simulink model "elevation_techo_PLANT"  (R2022a)
settings: Solver=VariableStepAuto  StartTime=0.0  StopTime=100.0  RelTol=1e-4
undefined symbols (not defined in the file or in its folder): fix_conset, JLret, JMret, Kket, Kvet
libraries: slctrlblks x1
settings Model: Creator=ohadformanair  LastModifiedBy=ohadformanair
settings SolverCC: ZeroCrossAlgorithm=Adaptive
settings DebuggingCC: IgnoredZcDiagnostic=none

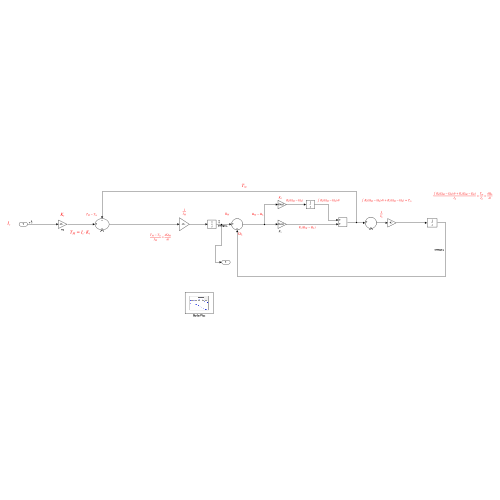
[thumbnail: Simulink's stored preview of the top-level diagram]
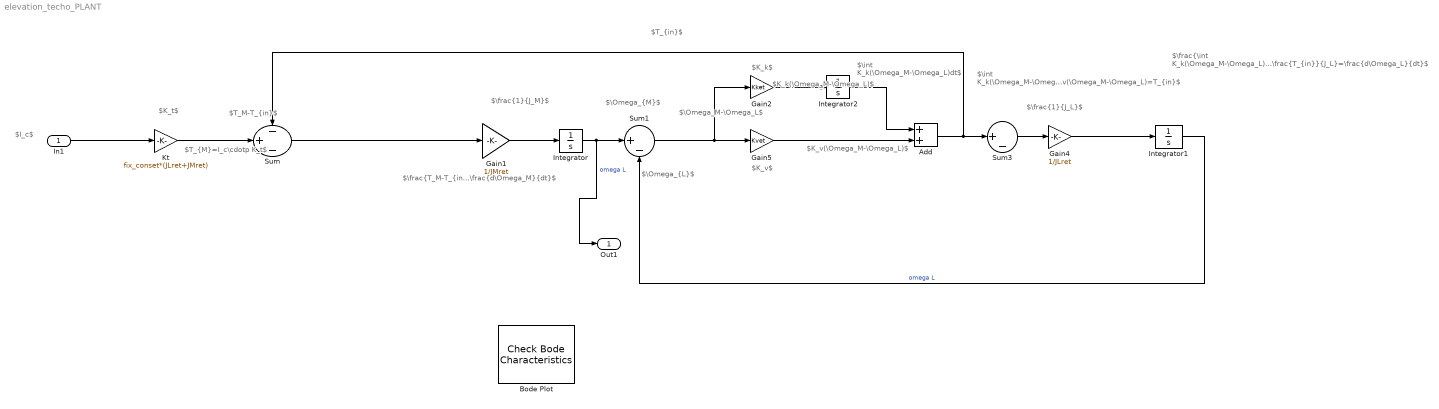
== system elevation_techo_PLANT ==
  note: $\Omega_{L}$
  note: $\frac{1}{J_L}$
  note: $K_v(\Omega_M-\Omega_L)$
  note: $T_{M}=I_c\cdotp K_t$
  note: $\frac{T_M-T_{in}}{J_M}=\frac{d\Omega_M}{dt}$
  note: $\int K_k(\Omega_M-\Omega_L)dt+K_v(\Omega_M-\Omega_L)=T_{in}$
  note: $I_c$
  note: $T_M-T_{in}$
  note: $K_k$
  note: $\Omega_M-\Omega_L$
  note: $\int K_k(\Omega_M-\Omega_L)dt$
  note: $K_k(\Omega_M-\Omega_L)$
  note: $\frac{1}{J_M}$
  note: $\frac{\int K_k(\Omega_M-\Omega_L)dt+K_v(\Omega_M-\Omega_L)}{J_L}=\frac{T_{in}}{J_L}=\frac{d\Omega_L}{dt}$
  note: $\Omega_{M}$
  note: $K_t$
  note: $K_v$
  note: $T_{in}$
  In1 : Inport
  Add : Sum
  Bode Plot : slctrlblks/Model Verification/Check Bode  Characteristics  InstantiateOnLoad=on  SaveOperatingPoints=off  LinearizationIOs={'/In1', 1, 'in', 'off', '';'/Integrator', 1, 'out', 'off', ''}  LinearizeAt=SnapshotTimes  SnapshotTimes=[0]  TriggerType=rising  SampleTime=auto  RateConversionMethod=zoh  PreWarpFreq=10  UseExactDelayModel=off  UseFullBlockNameLabels=off  UseBusSignalLabels=off  enabled=on  stopWhenAssertionFail=off  export=off  ViewDlgPos=[100 200 510 390]  OpenViewOnLoad=off  LaunchViewOnOpen=off  FrequencyUnits=Hz  MagnitudeUnits=dB  PhaseUnits=deg  TimeUnits=seconds  EnableUpperBound=off  UpperBoundFrequencies=[]  UpperBoundMagnitudes=[]  EnableLowerBound=off  LowerBoundFrequencies=[]  LowerBoundMagnitudes=[]
  Gain1 : Gain  Gain=1/JMret
  Gain2 : Gain  Gain=Kket
  Gain4 : Gain  Gain=1/JLret
  Gain5 : Gain  Gain=Kvet
  Integrator : Integrator
  Integrator1 : Integrator
  Integrator2 : Integrator
  Kt : Gain  Gain=fix_conset*(JLret+JMret)
  Sum : Sum  Inputs=-+-
  Sum1 : Sum  Inputs=|+-
  Sum3 : Sum  Inputs=|+-
  Out1 : Outport
  wires:
  Gain1/1 -> Integrator/1
  Kt/1 -> Sum/2
  Gain2/1 -> Integrator2/1
  Sum/1 -> Gain1/1
  Add/1 -> Sum3/1, Sum/1
  Integrator1/1 -> Sum1/2  "omega L"
  Gain4/1 -> Integrator1/1
  Integrator2/1 -> Add/1
  Gain5/1 -> Add/2
  Sum1/1 -> Gain5/1, Gain2/1
  Sum3/1 -> Gain4/1
  Integrator/1 -> Out1/1, Sum1/1  "omega L"
  In1/1 -> Kt/1
